simulink model "Bezout_311"  (Simulink 7.3)
settings: Solver=ode5  StartTime=0.0  StopTime=1000  FixedStep=0.01  RelTol=1e-3
StopFcn:
  | subplot(211);
  | plot(Data.time,Data.signals(1).values(:,1),'r',Data.time,Data.signals(1).values(:,2),'b')
  | subplot(212);
  | plot(Data.time,Data.signals(2).values(:,1),'b')
values from neighbouring files (symbols this model uses):
  a1 = -p-conj(p)    [ARMA_vs_Correlogram.m]    (also in AR_vs_Correlogram.m; tn_nn1.m = 1; tn_nn2.m = 1./p1)
undefined symbols (not defined in the file or in its folder): a0, k
libraries: simulink x1
settings Model: Creator=Minh-Map-Vu  LastModifiedBy=nthuy
settings DataIOCC: SignalLoggingName=sigsOut
settings DebuggingCC: SaveWithParameterizedLinksMsg=none  SignalResolutionControl=TryResolveAllWithWarning  SolverPrmCheckMsg=none  MultiTaskDSMMsg=warning  MultiTaskCondExecSysMsg=none  StrictBusMsg=None
settings HardwareCC: TargetUnknown=on
settings RTWCC: IncludeERTFirstTime=on

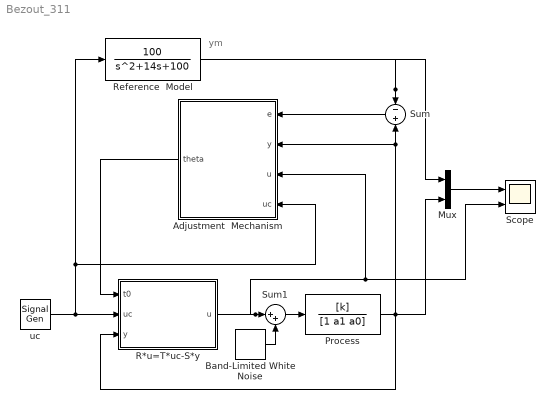
== system Bezout_311 ==
  note: ym
  Adjustment  Mechanism : Subsystem
  Band-Limited White Noise : simulink/Sources/Band-Limited White Noise  SystemSampleTime=-1  Cov=[0.1]  Ts=0.01  seed=[23341]
  Mux : Mux  Inputs=2
  Process : TransferFcn  Numerator=[k]  Denominator=[1 a1 a0]
  R*u=T*uc-S*y : Subsystem
  Reference  Model : TransferFcn  Numerator=[100]  Denominator=[1 14 100]
  Scope : Scope  NumInputPorts=2
      settings: TimeRange=100  YMin=-1.2~-5  YMax=1.2~5  SaveName=Data
  Sum : Sum  Inputs=-+  SaturateOnIntegerOverflow=on
  Sum1 : Sum  Inputs=|++  OutDataType=fixdt(1, 16)  OutScaling=2^0
  uc : SignalGenerator  WaveForm=square  Frequency=1/20
  wires:
  Mux/1 -> Scope/1
  uc/1 -> R*u=T*uc-S*y/2(uc), Reference  Model/1, Adjustment  Mechanism/4(uc)
  Reference  Model/1 -> Sum/1, Mux/1
  Sum/1 -> Adjustment  Mechanism/1(e)
  Adjustment  Mechanism/1(theta) -> R*u=T*uc-S*y/1(t0)
  R*u=T*uc-S*y/1(u) -> Adjustment  Mechanism/3(u), Scope/2, Sum1/1
  Process/1 -> Sum/2, Adjustment  Mechanism/2(y), R*u=T*uc-S*y/3(y), Mux/2
  Sum1/1 -> Process/1
  Band-Limited White Noise/1 -> Sum1/2

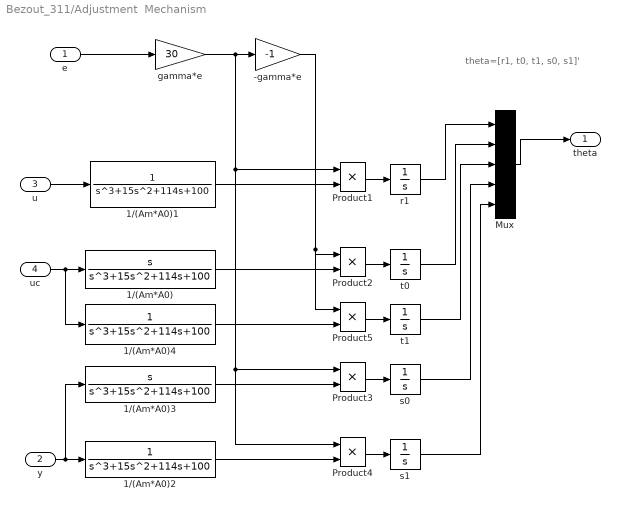
== system Bezout_311/Adjustment  Mechanism ==
  note: theta=[r1, t0, t1, s0, s1]'
  e : Inport
  y : Inport  Port=2
  u : Inport  Port=3
  uc : Inport  Port=4
  -gamma*e : Gain  Gain=-1  SaturateOnIntegerOverflow=on  OutDataTypeStr=Inherit: Same as input  ParamDataTypeStr=Inherit: Same as input
  1/(Am*A0) : TransferFcn  Numerator=[1 0]  Denominator=[1 15 114 100]
  1/(Am*A0)1 : TransferFcn  Numerator=1  Denominator=[1 15 114 100]
  1/(Am*A0)2 : TransferFcn  Numerator=1  Denominator=[1 15 114 100]
  1/(Am*A0)3 : TransferFcn  Numerator=[1 0]  Denominator=[1 15 114 100]
  1/(Am*A0)4 : TransferFcn  Numerator=1  Denominator=[1 15 114 100]
  Mux : Mux  Inputs=5
  Product{1..5} (5 alike) : Product  SaturateOnIntegerOverflow=on  OutDataTypeStr=Inherit: Same as first input
  gamma*e : Gain  Gain=30  SaturateOnIntegerOverflow=on  OutDataTypeStr=Inherit: Same as input  ParamDataTypeStr=Inherit: Same as input
  r1 : Integrator  InitialCondition=20*rand  LimitOutput=on  LowerSaturationLimit=0
  s0 : Integrator  InitialCondition=20*rand  LimitOutput=on  LowerSaturationLimit=0
  s1 : Integrator  InitialCondition=20*rand  LimitOutput=on  LowerSaturationLimit=0
  t0 : Integrator  InitialCondition=20*rand  LimitOutput=on  LowerSaturationLimit=0
  t1 : Integrator  InitialCondition=20*rand  LimitOutput=on  LowerSaturationLimit=0
  theta : Outport
  wires:
  Mux/1 -> theta/1
  uc/1 -> 1/(Am*A0)/1, 1/(Am*A0)4/1
  e/1 -> gamma*e/1
  y/1 -> 1/(Am*A0)2/1, 1/(Am*A0)3/1
  u/1 -> 1/(Am*A0)1/1
  gamma*e/1 -> -gamma*e/1, Product1/1, Product4/1, Product3/1
  Product1/1 -> r1/1
  1/(Am*A0)1/1 -> Product1/2
  1/(Am*A0)/1 -> Product2/2
  Product2/1 -> t0/1
  -gamma*e/1 -> Product2/1, Product5/1
  Product3/1 -> s0/1
  Product4/1 -> s1/1
  1/(Am*A0)2/1 -> Product4/2
  1/(Am*A0)3/1 -> Product3/2
  r1/1 -> Mux/1
  t0/1 -> Mux/2
  s1/1 -> Mux/5
  s0/1 -> Mux/4
  Product5/1 -> t1/1
  1/(Am*A0)4/1 -> Product5/2
  t1/1 -> Mux/3

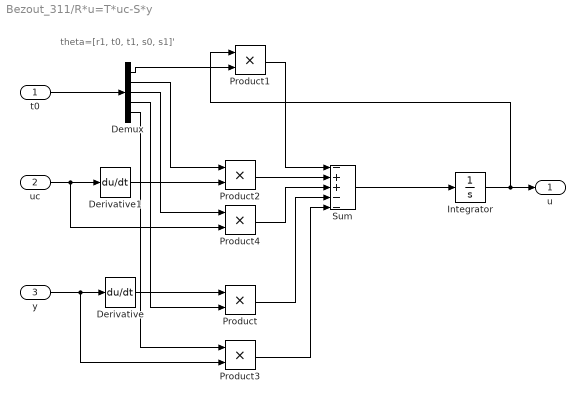
== system Bezout_311/R*u=T*uc-S*y ==
  note: theta=[r1, t0, t1, s0, s1]'
  t0 : Inport
  uc : Inport  Port=2
  y : Inport  Port=3
  Demux : Demux  Outputs=5
  Derivative : Derivative
  Derivative1 : Derivative
  Integrator : Integrator
  Product{,1..4} (5 alike) : Product  SaturateOnIntegerOverflow=on  OutDataTypeStr=Inherit: Same as first input
  Sum : Sum  Inputs=-++--  SaturateOnIntegerOverflow=on
  u : Outport
  wires:
  Integrator/1 -> u/1, Product1/1
  y/1 -> Derivative/1, Product3/2
  Derivative/1 -> Product/1
  t0/1 -> Demux/1
  uc/1 -> Derivative1/1, Product4/2
  Product2/1 -> Sum/2
  Product1/1 -> Sum/1
  Sum/1 -> Integrator/1
  Demux/1 -> Product1/2
  Demux/2 -> Product2/1
  Product3/1 -> Sum/5
  Product/1 -> Sum/4
  Derivative1/1 -> Product2/2
  Product4/1 -> Sum/3
  Demux/5 -> Product3/1
  Demux/4 -> Product/2
  Demux/3 -> Product4/1
